simulink model "testrig_AxleTA4Watts"  (R2025b)
settings: Solver=ode23t  StartTime=0.0  StopTime=10.0  RelTol=1e-3  AbsTol=1e-3  EnableMultiTasking=on
PostLoadFcn:
  | sm_car_load_vehicle_data(bdroot,'231');
undefined symbols (not defined in the file): Vehicle, X, Y, Z
libraries: sm_lib x15, fl_lib x8, Damper_Element x2, Spring_Element x2, Susp_AxleTA4Watts x1, nesl_utility x1
Description:
  | Testrig for Solid Axle, Four Trailing Arm, Watts Link Suspension
  | 
  | Copyright 2018-2025 The MathWorks, Inc.
settings Model: VariantFading=off  Creator=smiller  LastModifiedBy=smiller
settings SolverCC: AutoScaleAbsTol=off  AlgebraicLoopSolver=TrustRegion
settings DataIOCC: LimitDataPoints=on  ReturnWorkspaceOutputs=off  SignalLoggingName=logsout_testrig_AxleTA4Watts
settings OptimizationCC: LifeSpan=inf
settings DebuggingCC: UnconnectedInputMsg=warning  UnconnectedOutputMsg=warning  UnconnectedLineMsg=warning  AllowSymbolicDim=off  SFUnexpectedBacktrackingDiag=warning  SFNoUnconditionalDefaultTransitionDiag=warning  SFExecutionAtInitializationDiag=none  ArithmeticOperatorsInVariantConditions=warning
settings ModelReferenceCC: EnableRefExpFcnMdlSchedulingChecks=on
settings SFSimCC: SimUseLocalCustomCode=off  CustomCodeUndefinedFunction=UseInterfaceOnly
settings RTWCC: RTWUseLocalCustomCode=off  GPUComputeCapability=3.5  DLArmComputeVersion=19.05
settings CodeAppCC: StateflowObjectComments=on
settings GRTTargetCC: TargetLangStandard=C89/C90 (ANSI)
settings ConfigComp: CovMetricSettings=dw  CovSaveCumulativeToWorkspaceVar=on  CovSaveSingleToWorkspaceVar=on  CovExternalEMLEnable=off  CovSFcnEnable=off
settings SimscapeCC: SimscapeNominalValues="[{\"value\":\"10\",\"unit\":\"V\"},{\"value\":\"1\",\"unit\":\"A\"},{\"value\":\"10\",\"unit\":\"N*m\"},{\"value\":\"10\",\"unit\":\"bar\"},{\"value\":\"100\",\"unit\":\"kJ/kg\"},{\"value\":\"1\",\"unit\":\"kW\"},{\"value\":\"300\",\"unit\":\"K\"},{\"value\":\"100\",\"unit\":\"cm^3/s\"},{\"value\":\"1\",\"unit\":\"kN\"},{\"value\":\"1\",\"unit\":\"g/cm^3\"},{\"value\":\"1\",\"unit\":\"l\"},{\"value\":\"1\",\"unit\":\"cm^2\"},{\"value\":\"60\",\"unit\":\"Hz\"}]"  SimscapeLogType=all  SimscapeLogName=simlog_testrig_AxleTA3  SimscapeLogLimitData=off  SimscapeLogDataHistory=10000.0
settings ConfigurationSet: Description=SimMechanics 2G
settings DiagnosticsConfigSet: SimMechanicsUnconnectedFramePorts=none  SimMechanicsConflictingReferenceFrames=none
settings ExplorerConfigSet: InternalSimMechanicsExplorerSettings="<ExplorerConfiguration><canonicalview>default</canonicalview><AnimationSetting><BasePlaybackSpeed>1.0</BasePlaybackSpeed><PlaybackSpeedFactor>1.0</PlaybackSpeedFactor></AnimationSetting><TilePanel><TileInfo><Tiles Columns=\"2\" Count=\"3\" Rows=\"2\"><Column Weight=\"0.4244\"/><Column Weight=\"0.5756\"/><Row Weight=\"0.4992\"/><Row Weight=\"0.5008\"/><Tile Height=\"2\" Width=\"1\" X=\"0\" Y=\"0\"/><Tile Height=\"1\" Width=\"1\" X=\"1\" Y=\"0\"/><Tile Height=\"1\" Width=\"1\" X=\"1\" Y=\"1\"/></Tiles></TileInfo><SceneInfo><SceneViewer><BGColor><R>1</R><G>1</G><B>1</B></BGColor><Camera><DoPerspective>off</DoPerspective><Position><X>0.552478174350915729</X><Y>-0.803945093768714147</Y><Z>1.32502797539261552</Z></Position><Center><X>0.0812867764930292336</X><Y>0.0151540971816948034</Y><Z>0.373221841276778488</Z></Center><Up><X>-0.368839640393352541</X><Y>0.60639690830076276</Y><Z>0.704443119973344745</Z></Up><ViewLimDist>1</ViewLimDist><YLim>1.05019854224089437</YLim><XLim>0.873694585561752501</XLim></Camera></SceneViewer><SceneViewer><BGColor><R>1</R><G>1</G><B>1</B></BGColor><Camera><DoPerspective>off</DoPerspective><Position><X>0.0192474230206069602</X><Y>0.00226632239327399527</Y><Z>2.4899249315669274</Z></Position><Center><X>0.0192474230206069602</X><Y>0.00226632239327399527</Y><Z>0.826695781607784674</Z></Center><Up><X>-0.999990402627246699</X><Y>-0.00438117032276797314</Y><Z>0</Z></Up><ViewLimDist>1</ViewLimDist><YLim>0.508295861926471582</YLim><XLim>1.16532602435983668</XLim></Camera></SceneViewer><SceneViewer><BGColor><R>1</R><G>1</G><B>1</B></BGColor><Camera><DoPerspective>off</DoPerspective><Position><X>0.182585918864573593</X><Y>-1.79252728458574717</Y><Z>0.406437226559380693</Z></Position><Center><X>0.182585918864573593</X><Y>0.0093803152648429533</Y><Z>0.406437226559380693</Z></Center><Up><X>0</X><Y>-0</Y><Z>1</Z></Up><ViewLimDist>1</ViewLimDist><YLim>0.57204496088982637</YLim><XLim>1.30776284260082121</XLim></Camera></SceneViewer></SceneInfo></TilePanel><MechEditorPanel><Cameras/><GfxPanelCameraMap/><VideoCreator><PlaybackSpeedRatio>1.0</PlaybackSpeedRatio><FrameRate>30</FrameRate><VideoFormat>MPEG-4</VideoFormat><FrameSize>auto</FrameSize></VideoCreator></MechEditorPanel></ExplorerConfiguration>"

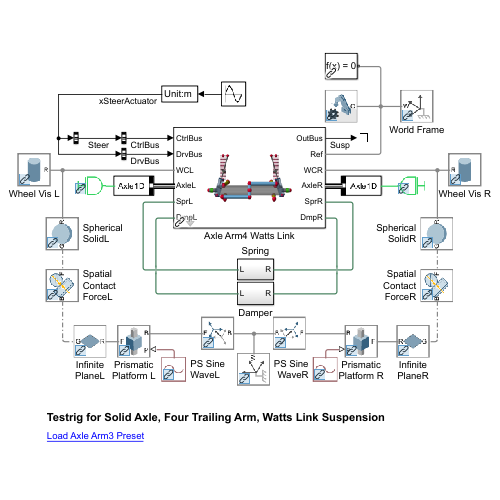
[thumbnail: Simulink's stored preview of the top-level diagram]
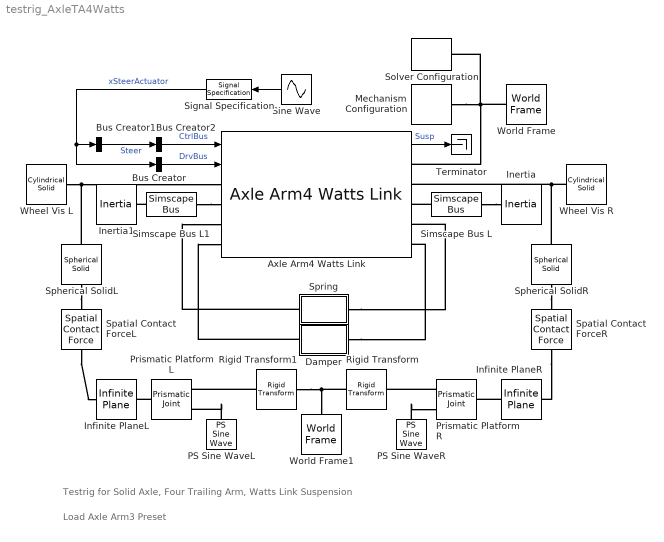
== system testrig_AxleTA4Watts ==
  note: Load Axle Arm3 Preset
  note: Testrig for Solid Axle, Four Trailing Arm, Watts Link Suspension
  Axle Arm4 Watts Link : Susp_AxleTA4Watts/Axle Arm4 Watts Link  VariantControl=LiveAxle  Init=Init.Axle2  hp_damper_top=Vehicle.Chassis.SuspA2.AxleTA4Watts.Damper.sTop.Value  hp_damper_bot=Vehicle.Chassis.SuspA2.AxleTA4Watts.Damper.sBottom.Value  hp_spring_top=Vehicle.Chassis.SuspA2.AxleTA4Watts.Spring.sTop.Value  hp_spring_bot=Vehicle.Chassis.SuspA2.AxleTA4Watts.Spring.sBottom.Value  hp_ua_body=Vehicle.Chassis.SuspA2.AxleTA4Watts.TrailingArmUpper.sBody.Value  hp_ua_axle=Vehicle.Chassis.SuspA2.AxleTA4Watts.TrailingArmUpper.sAxle.Value  hp_la_body=Vehicle.Chassis.SuspA2.AxleTA4Watts.TrailingArmLower.sBody.Value  hp_la_axle=Vehicle.Chassis.SuspA2.AxleTA4Watts.TrailingArmLower.sAxle.Value  hp_wattsu_body=Vehicle.Chassis.SuspA2.AxleTA4Watts.WattsLinkUpper.sBody.Value  hp_wattsu_pivot=Vehicle.Chassis.SuspA2.AxleTA4Watts.WattsLinkUpper.sPivot.Value  hp_wattsl_body=Vehicle.Chassis.SuspA2.AxleTA4Watts.WattsLinkLower.sBody.Value  hp_wattsl_pivot=Vehicle.Chassis.SuspA2.AxleTA4Watts.WattsLinkLower.sPivot.Value  hp_wattsp_axle=Vehicle.Chassis.SuspA2.AxleTA4Watts.WattsLinkPivot.sAxle.Value  hp_axle_cg=Vehicle.Chassis.SuspA2.AxleTA4Watts.Axle.sCG.Value  hp_whl_ctr=Vehicle.Chassis.SuspA2.AxleTA4Watts.Axle.sWheelCentre.Value  hp_chassis_bumpstop=Vehicle.Chassis.SuspA2.AxleTA4Watts.Bumpstop.sChassis.Value  hp_axle_bumpstop=Vehicle.Chassis.SuspA2.AxleTA4Watts.Bumpstop.sAxle.Value  axle_mass=Vehicle.Chassis.SuspA2.AxleTA4Watts.Axle.m.Value  stub_axle_len=Vehicle.Chassis.SuspA2.AxleTA4Watts.StubAxle.xAxle.Value  stub_axle_mass=Vehicle.Chassis.SuspA2.AxleTA4Watts.StubAxle.m.Value  axle_whlc_to_bearing=Vehicle.Chassis.SuspA2.AxleTA4Watts.Axle.xWCtoBearing.Value  ua_mass=Vehicle.Chassis.SuspA2.AxleTA4Watts.TrailingArmUpper.m.Value  la_mass=Vehicle.Chassis.SuspA2.AxleTA4Watts.TrailingArmLower.m.Value  wattsu_mass=Vehicle.Chassis.SuspA2.AxleTA4Watts.WattsLinkUpper.m.Value  wattsl_mass=Vehicle.Chassis.SuspA2.AxleTA4Watts.WattsLinkLower.m.Value  wattsp_mass=Vehicle.Chassis.SuspA2.AxleTA4Watts.WattsLinkLower.m.Value  clr_conn_rod=Visual.hp.clr  opc_conn_rod=Visual.hp.opc  size_conn_rod=Visual.hp.rad  clr_rod=Visual.UpperArm.clr  opc_rod=Visual.part.opc  radius_rod=Visual.UpperArm.rad  clr_link=Visual.Pushrod.clr  opc_link=Visual.part.opc  radius_link=Visual.Pushrod.rad  axle_clr=[0.5 0.5 0.5]  axle_opc=Visual.part.opc  clr_stub_axle=Visual.Axle.clr  opc_stub_axle=Visual.part.opc  rad_stub_axle=Visual.Axle.rad  shock_pist_mass=Vehicle.Chassis.SuspA2.AxleTA4Watts.Damper.mPiston.Value  shock_cyl_mass=Vehicle.Chassis.SuspA2.AxleTA4Watts.Damper.mCylinder.Value  shock_xmax=Vehicle.Chassis.SuspA2.AxleTA4Watts.Endstop.xMax.Value  shock_xmin=Vehicle.Chassis.SuspA2.AxleTA4Watts.Endstop.xMin.Value  spring_mass=Vehicle.Chassis.SuspA2.AxleTA4Watts.Spring.m.Value  Bumpstop_Type=Vehicle.Chassis.SuspA2.AxleTA4Watts.Bumpstop.class.Value  bumpstop_height=Vehicle.Chassis.SuspA2.AxleTA4Watts.Bumpstop.xHeight.Value  bumpstop_k=Vehicle.Chassis.SuspA2.AxleTA4Watts.Bumpstop.K.Value  bumpstop_d=Vehicle.Chassis.SuspA2.AxleTA4Watts.Bumpstop.d.Value  bumpstop_xTrans=Vehicle.Chassis.SuspA2.AxleTA4Watts.Bumpstop.xTransition.Value  bumpstop_ptcld=Vehicle.Chassis.SuspA2.AxleTA4Watts.Bumpstop.sPointCloud.Value
  Bus Creator : BusCreator  Inputs=1
  Bus Creator1 : BusCreator  Inputs=1
  Bus Creator2 : BusCreator  Inputs=1
  Damper : Subsystem
  Inertia : fl_lib/Mechanical/Rotational Elements/Inertia  inertia=1 kg*m^2  num_ports=foundation.enum.numPorts2.one  w_specify=on  w_priority=None  w=0 rad/s  w_nominal_specify=off  w_nominal_value=1  w_nominal_unit=rad/s  t_specify=off  t_priority=None  t=0 N*m  t_nominal_specify=off  t_nominal_value=1  t_nominal_unit=N*m
  Inertia1 : fl_lib/Mechanical/Rotational Elements/Inertia  inertia=1 kg*m^2  num_ports=foundation.enum.numPorts2.one  w_specify=on  w_priority=None  w=0 rad/s  w_nominal_specify=off  w_nominal_value=1  w_nominal_unit=rad/s  t_specify=off  t_priority=None  t=0 N*m  t_nominal_specify=off  t_nominal_value=1  t_nominal_unit=N*m
  Infinite PlaneL : sm_lib/Curves and Surfaces/Infinite Plane  GraphicType=Rectangle  GraphicPlaneWidth=0.3  GraphicPlaneWidthUnits=m  GraphicPlaneHeight=0.3  GraphicPlaneHeightUnits=m  GraphicVisPropType=SimpleVisualProperties  GraphicDiffuseColor=[0.5 0.5 0.5]  GraphicOpacity=0.5  GraphicSpecularColor=[0.5 0.5 0.5 1.0]  GraphicAmbientColor=[0.15 0.15 0.15 1.0]  GraphicEmissiveColor=[0.0 0.0 0.0 1.0]  GraphicShininess=75
  Infinite PlaneR : sm_lib/Curves and Surfaces/Infinite Plane  GraphicType=Rectangle  GraphicPlaneWidth=0.3  GraphicPlaneWidthUnits=m  GraphicPlaneHeight=0.3  GraphicPlaneHeightUnits=m  GraphicVisPropType=SimpleVisualProperties  GraphicDiffuseColor=[0.5 0.5 0.5]  GraphicOpacity=0.5  GraphicSpecularColor=[0.5 0.5 0.5 1.0]  GraphicAmbientColor=[0.15 0.15 0.15 1.0]  GraphicEmissiveColor=[0.0 0.0 0.0 1.0]  GraphicShininess=75
  Mechanism Configuration : sm_lib/Utilities/Mechanism Configuration  UniformGravity=Constant  GravityVector=[0 0 -9.80665]  GravityVectorUnits=m/s^2  LinearizationDelta=0.001  JointModeTransitionNonlinearIterations=2
  PS Sine WaveL : fl_lib/Physical Signals/Sources/PS Sine Wave  amplitude=0.05 m  bias=0 m  frequency_spec=foundation.enum.frequencySpec.frequencySI  frequency_SI=4/3 Hz  frequency_angular=1 rad/s  phase=pi rad
      settings: InternalSimscapePortConfiguration="{\"Bottom\":[],\"Left\":[],\"Right\":[{\"id\":\"O\",\"label\":\"\",\"type\":\"output\"}],\"Top\":[]}"
  PS Sine WaveR : fl_lib/Physical Signals/Sources/PS Sine Wave  amplitude=0.1 m  bias=0 m  frequency_spec=foundation.enum.frequencySpec.frequencySI  frequency_SI=1 Hz  frequency_angular=1 rad/s  phase=0 rad
      settings: InternalSimscapePortConfiguration="{\"Bottom\":[],\"Left\":[],\"Right\":[{\"id\":\"O\",\"label\":\"\",\"type\":\"output\"}],\"Top\":[]}"
  Prismatic Platform L : sm_lib/Joints/Prismatic Joint  JointMode=Normal  CompositeWrenchDir=FollowerOnBase  CompositeWrenchFrame=BaseFrame  SenseConstraintForce=off  SenseConstraintTorque=off  SenseTotalForce=off  SenseTotalTorque=off  PositionTargetSpecify=off  PositionTargetPriority=High  PositionTargetValue=0  PositionTargetValueUnits=m  VelocityTargetSpecify=off  VelocityTargetPriority=High  VelocityTargetValue=0  VelocityTargetValueUnits=m/s  EquilibriumPosition=0  EquilibriumPositionUnits=m  SpringStiffness=0  SpringStiffnessUnits=N/m  DampingCoefficient=0  DampingCoefficientUnits=N/(m/s)  LowerLimitSpecify=off  LowerLimitBound=-1  LowerLimitBoundUnits=m  LowerLimitStiffness=1e6  LowerLimitStiffnessUnits=N/m  LowerLimitDamping=1e3  LowerLimitDampingUnits=N/(m/s)  LowerLimitTransitionRegionWidth=1e-4  LowerLimitTransitionRegionWidthUnits=m  UpperLimitSpecify=off  UpperLimitBound=1  UpperLimitBoundUnits=m  UpperLimitStiffness=1e6  UpperLimitStiffnessUnits=N/m  UpperLimitDamping=1e3  UpperLimitDampingUnits=N/(m/s)  UpperLimitTransitionRegionWidth=1e-4  UpperLimitTransitionRegionWidthUnits=m  TorqueActuationMode=ComputedTorque  MotionActuationMode=InputMotion  SensePosition=off  SenseVelocity=off  SenseAcceleration=off  SenseTorqueForce=off  SenseLowerLimitTorqueForce=off  SenseUpperLimitTorqueForce=off
  Prismatic Platform R : sm_lib/Joints/Prismatic Joint  JointMode=Normal  CompositeWrenchDir=FollowerOnBase  CompositeWrenchFrame=BaseFrame  SenseConstraintForce=off  SenseConstraintTorque=off  SenseTotalForce=off  SenseTotalTorque=off  PositionTargetSpecify=off  PositionTargetPriority=High  PositionTargetValue=0  PositionTargetValueUnits=m  VelocityTargetSpecify=off  VelocityTargetPriority=High  VelocityTargetValue=0  VelocityTargetValueUnits=m/s  EquilibriumPosition=0  EquilibriumPositionUnits=m  SpringStiffness=0  SpringStiffnessUnits=N/m  DampingCoefficient=0  DampingCoefficientUnits=N/(m/s)  LowerLimitSpecify=off  LowerLimitBound=-1  LowerLimitBoundUnits=m  LowerLimitStiffness=1e6  LowerLimitStiffnessUnits=N/m  LowerLimitDamping=1e3  LowerLimitDampingUnits=N/(m/s)  LowerLimitTransitionRegionWidth=1e-4  LowerLimitTransitionRegionWidthUnits=m  UpperLimitSpecify=off  UpperLimitBound=1  UpperLimitBoundUnits=m  UpperLimitStiffness=1e6  UpperLimitStiffnessUnits=N/m  UpperLimitDamping=1e3  UpperLimitDampingUnits=N/(m/s)  UpperLimitTransitionRegionWidth=1e-4  UpperLimitTransitionRegionWidthUnits=m  TorqueActuationMode=ComputedTorque  MotionActuationMode=InputMotion  SensePosition=off  SenseVelocity=off  SenseAcceleration=off  SenseTorqueForce=off  SenseLowerLimitTorqueForce=off  SenseUpperLimitTorqueForce=off
  Rigid Transform : sm_lib/Frames and Transforms/Rigid Transform  RotationMethod=None  FollAlignAxisA=+X  BaseAlignAxisA=+Y  FollAlignAxisB=+Y  BaseAlignAxisB=+Z  RotationStandardAxis=+Z  RotationAngle=0  RotationAngleUnits=deg  RotationArbitraryAxis=[0 0 1]  RotationSequenceAxes=FollowerAxes  RotationSequence=XYX  RotationSequenceAngles=[0 0 0]  RotationSequenceAnglesUnits=deg  RotationMatrix=[1 0 0;0 1 0;0 0 1]  Quaternion=[1 0 0 0]  TranslationMethod=Cartesian  TranslationCartesianOffset=Vehicle.Chassis.SuspA2.AxleTA4Watts.Axle.sWheelCentre.Value.*[1 -1 0]  TranslationCartesianOffsetUnits=m  TranslationStandardAxis=+Z  TranslationStandardOffset=0  TranslationStandardOffsetUnits=m  TranslationROffset=0  TranslationROffsetUnits=m  TranslationThetaOffset=0  TranslationThetaOffsetUnits=deg  TranslationZOffset=0  TranslationZOffsetUnits=m
  Rigid Transform1 : sm_lib/Frames and Transforms/Rigid Transform  RotationMethod=None  FollAlignAxisA=+X  BaseAlignAxisA=+Y  FollAlignAxisB=+Y  BaseAlignAxisB=+Z  RotationStandardAxis=+Z  RotationAngle=0  RotationAngleUnits=deg  RotationArbitraryAxis=[0 0 1]  RotationSequenceAxes=FollowerAxes  RotationSequence=XYX  RotationSequenceAngles=[0 0 0]  RotationSequenceAnglesUnits=deg  RotationMatrix=[1 0 0;0 1 0;0 0 1]  Quaternion=[1 0 0 0]  TranslationMethod=Cartesian  TranslationCartesianOffset=Vehicle.Chassis.SuspA2.AxleTA4Watts.Axle.sWheelCentre.Value.*[1 1 0]  TranslationCartesianOffsetUnits=m  TranslationStandardAxis=+Z  TranslationStandardOffset=0  TranslationStandardOffsetUnits=m  TranslationROffset=0  TranslationROffsetUnits=m  TranslationThetaOffset=0  TranslationThetaOffsetUnits=deg  TranslationZOffset=0  TranslationZOffsetUnits=m
  Signal Specification : SignalSpecification  Unit=m
  Simscape Bus L : SimscapeBus  HierarchyStrings=Axle1D
  Simscape Bus L1 : SimscapeBus  HierarchyStrings=Axle1D
  Sine Wave : Sin  Amplitude=0.1  Frequency=pi/4  SampleTime=0
  Solver Configuration : nesl_utility/Solver Configuration  PhysicalDomain=network_engine_domain  SubClassName=solver  LeftPortType=input  RightPortType=generic  Tones=[]  Harmonics=[]  SimulateNoise=off  Profile=off  UseLocalSampling=off  EnableSwitchedLinearOptims=on  FrequencyDomain=off  UseCCode=off  RelTol=0.001  AbsTol=1e-06  MinStep=1e-09  ToWorkspace=off  RevertToSquareIcSolve=off  NumHomotopyIterations=100  PhasorMode=off  PhasorModeNumHarmonics=1  ConsistencySolver=NEWTON_FTOL  IndexReductionMethod=DerivativeReplacement  DoDC=off  ResidualTolerance=1e-09  ConsistencyTolSource=GLOBAL  ConsistencyAbsTol=0.001  ConsistencyRelTol=0.001  ConsistencyTolFactor=0.001  UseLocalSolver=off  LocalSolverChoice=NE_BACKWARD_EULER_ADVANCER  ResolveIndetEquations=on  FunctionEvalNumThread=1  LocalSolverSampleTime=0.001  DoFixedCost=off  MaxNonlinIter=3  MaxModeIter=2  ComputeImpulses=off  ImpulseIterations=2  LinearAlgebra=Sparse  LinearAlgebraNumThread=0  EquationFormulation=NE_TIME_EF  DelaysMemoryBudget=1024  AutomaticFiltering=on  FilteringTimeConstant=0.001  PartitionStorageMethod=AS_NEEDED  PartitionMemoryBudget=1024  PartitionMethod=FAST  MultibodyUseLocalSolver=off  MultibodyLocalSolverChoice=ODE1  MultibodyLocalSolverSampleTime=0.001
  Spatial Contact ForceL : sm_lib/Forces and Torques/Spatial Contact Force  SenseSeparationDistance=off  NormalForceType=SmoothSpringDamper  NormalStiffness=1e6  NormalStiffnessUnits=N/m  NormalDamping=1e3  NormalDampingUnits=N/(m/s)  NormalTransitionRegionWidth=1e-4  NormalTransitionRegionWidthUnits=m  FrictionType=None  CoefficientOfStaticFriction=0.5  CoefficientOfDynamicFriction=0.3  FrictionalCriticalVelocity=1e-3  FrictionalCriticalVelocityUnits=m/s  SenseContactSignal=off  SensePenetrationDepth=off  SenseNormalVelocity=off  SenseTangentialVelocity=off  SensingForceTorqueDirection=BaseOnFollower  SensingForceTorqueResolutionFrame=ContactFrame  SenseNormalForce=off  SenseNormalForceMagnitude=off  SenseNormalTorque=off  SenseFrictionalForce=off  SenseFrictionalForceMagnitude=off  SenseFrictionalTorque=off  SenseTotalForce=off  SenseTotalTorque=off  SenseContactBaseRotation=off  SenseContactBaseTranslation=off  SenseContactFollowerRotation=off  SenseContactFollowerTranslation=off  ZeroCrossDetectContactStartAndEnd=off
  Spatial Contact ForceR : sm_lib/Forces and Torques/Spatial Contact Force  SenseSeparationDistance=off  NormalForceType=SmoothSpringDamper  NormalStiffness=1e6  NormalStiffnessUnits=N/m  NormalDamping=1e3  NormalDampingUnits=N/(m/s)  NormalTransitionRegionWidth=1e-4  NormalTransitionRegionWidthUnits=m  FrictionType=None  CoefficientOfStaticFriction=0.5  CoefficientOfDynamicFriction=0.3  FrictionalCriticalVelocity=1e-3  FrictionalCriticalVelocityUnits=m/s  SenseContactSignal=off  SensePenetrationDepth=off  SenseNormalVelocity=off  SenseTangentialVelocity=off  SensingForceTorqueDirection=BaseOnFollower  SensingForceTorqueResolutionFrame=ContactFrame  SenseNormalForce=off  SenseNormalForceMagnitude=off  SenseNormalTorque=off  SenseFrictionalForce=off  SenseFrictionalForceMagnitude=off  SenseFrictionalTorque=off  SenseTotalForce=off  SenseTotalTorque=off  SenseContactBaseRotation=off  SenseContactBaseTranslation=off  SenseContactFollowerRotation=off  SenseContactFollowerTranslation=off  ZeroCrossDetectContactStartAndEnd=off
  Spherical SolidL : sm_lib/Body Elements/Spherical Solid  SphereRadius=Vehicle.Chassis.SuspA2.AxleTA4Watts.Axle.sWheelCentre.Value(3)  SphereRadiusUnits=m  ExportEntireGeometry=on  InertiaType=CalculateFromGeometry  BasedOnType=Density  Density=0  DensityUnits=kg/m^3  Mass=1  MassUnits=kg  CenterOfMass=[0 0 0]  CenterOfMassUnits=m  MomentsOfInertia=[1 1 1]  MomentsOfInertiaUnits=kg*m^2  ProductsOfInertia=[0 0 0]  ProductsOfInertiaUnits=kg*m^2  GraphicType=None  MarkerShape=Sphere  MarkerSize=10  GraphicVisPropType=SimpleVisualProperties  GraphicDiffuseColor=[1.0 0.0 0.2]  GraphicOpacity=0.5  GraphicSpecularColor=[0.5 0.5 0.5 1.0]  GraphicAmbientColor=[0.15 0.15 0.15 1.0]  GraphicEmissiveColor=[0.0 0.0 0.0 1.0]  GraphicShininess=75  DoExposeReferenceFrame=on  SerializedFrames=<Frames/>
  Spherical SolidR : sm_lib/Body Elements/Spherical Solid  SphereRadius=Vehicle.Chassis.SuspA2.AxleTA4Watts.Axle.sWheelCentre.Value(3)  SphereRadiusUnits=m  ExportEntireGeometry=on  InertiaType=CalculateFromGeometry  BasedOnType=Density  Density=0  DensityUnits=kg/m^3  Mass=1  MassUnits=kg  CenterOfMass=[0 0 0]  CenterOfMassUnits=m  MomentsOfInertia=[1 1 1]  MomentsOfInertiaUnits=kg*m^2  ProductsOfInertia=[0 0 0]  ProductsOfInertiaUnits=kg*m^2  GraphicType=None  MarkerShape=Sphere  MarkerSize=10  GraphicVisPropType=SimpleVisualProperties  GraphicDiffuseColor=[1.0 0.0 0.2]  GraphicOpacity=0.5  GraphicSpecularColor=[0.5 0.5 0.5 1.0]  GraphicAmbientColor=[0.15 0.15 0.15 1.0]  GraphicEmissiveColor=[0.0 0.0 0.0 1.0]  GraphicShininess=75  DoExposeReferenceFrame=on  SerializedFrames=<Frames/>
  Spring : Subsystem
  Terminator : Terminator
  Wheel Vis L : sm_lib/Body Elements/Cylindrical Solid  CylinderRadius=Vehicle.Chassis.SuspA2.AxleTA4Watts.Axle.sWheelCentre.Value(3)  CylinderRadiusUnits=m  CylinderLength=0.235  CylinderLengthUnits=m  ExportEntireGeometry=off  InertiaType=CalculateFromGeometry  BasedOnType=Density  Density=1000  DensityUnits=kg/m^3  Mass=1  MassUnits=kg  CenterOfMass=[0 0 0]  CenterOfMassUnits=m  MomentsOfInertia=[1 1 1]  MomentsOfInertiaUnits=kg*m^2  ProductsOfInertia=[0 0 0]  ProductsOfInertiaUnits=kg*m^2  GraphicType=FromGeometry  MarkerShape=Sphere  MarkerSize=10  GraphicVisPropType=SimpleVisualProperties  GraphicDiffuseColor=[0.5 0.5 0.5]  GraphicOpacity=0.3  GraphicSpecularColor=[0.5 0.5 0.5 1.0]  GraphicAmbientColor=[0.15 0.15 0.15 1.0]  GraphicEmissiveColor=[0.0 0.0 0.0 1.0]  GraphicShininess=75  DoExposeReferenceFrame=on  SerializedFrames=<Frames/>
  Wheel Vis R : sm_lib/Body Elements/Cylindrical Solid  CylinderRadius=Vehicle.Chassis.SuspA2.AxleTA4Watts.Axle.sWheelCentre.Value(3)  CylinderRadiusUnits=m  CylinderLength=0.235  CylinderLengthUnits=m  ExportEntireGeometry=off  InertiaType=CalculateFromGeometry  BasedOnType=Density  Density=1000  DensityUnits=kg/m^3  Mass=1  MassUnits=kg  CenterOfMass=[0 0 0]  CenterOfMassUnits=m  MomentsOfInertia=[1 1 1]  MomentsOfInertiaUnits=kg*m^2  ProductsOfInertia=[0 0 0]  ProductsOfInertiaUnits=kg*m^2  GraphicType=FromGeometry  MarkerShape=Sphere  MarkerSize=10  GraphicVisPropType=SimpleVisualProperties  GraphicDiffuseColor=[0.5 0.5 0.5]  GraphicOpacity=0.3  GraphicSpecularColor=[0.5 0.5 0.5 1.0]  GraphicAmbientColor=[0.15 0.15 0.15 1.0]  GraphicEmissiveColor=[0.0 0.0 0.0 1.0]  GraphicShininess=75  DoExposeReferenceFrame=on  SerializedFrames=<Frames/>
  World Frame : sm_lib/Frames and Transforms/World Frame
  World Frame1 : sm_lib/Frames and Transforms/World Frame
  wires:
  Sine Wave/1 -> Signal Specification/1
  Signal Specification/1 -> Bus Creator/1, Bus Creator1/1  "xSteerActuator"
  Bus Creator/1 -> Axle Arm4 Watts Link/2  "DrvBus"
  Bus Creator1/1 -> Bus Creator2/1  "Steer"
  Axle Arm4 Watts Link/1 -> Terminator/1  "Susp"
  Bus Creator2/1 -> Axle Arm4 Watts Link/1  "CtrlBus"
  connections:
  Wheel Vis L/RConn1 -- Spherical SolidL/RConn1 -- Axle Arm4 Watts Link/LConn1
  Simscape Bus L/LConn1 -- Inertia/LConn1
  Simscape Bus L1/LConn1 -- Inertia1/LConn1
  Wheel Vis R/RConn1 -- Spherical SolidR/RConn1 -- Axle Arm4 Watts Link/RConn2
  Spherical SolidR/LConn1 -- Spatial Contact ForceR/RConn1
  Rigid Transform/LConn1 -- Rigid Transform1/LConn1 -- World Frame1/RConn1
  Spherical SolidL/LConn1 -- Spatial Contact ForceL/RConn1
  Spatial Contact ForceR/LConn1 -- Infinite PlaneR/RConn1
  Spatial Contact ForceL/LConn1 -- Infinite PlaneL/RConn1
  Infinite PlaneR/LConn1 -- Prismatic Platform R/RConn1
  Prismatic Platform L/RConn1 -- Infinite PlaneL/LConn1
  PS Sine WaveR/RConn1 -- Prismatic Platform R/LConn2
  PS Sine WaveL/RConn1 -- Prismatic Platform L/LConn2
  Prismatic Platform R/LConn1 -- Rigid Transform/RConn1
  Rigid Transform1/RConn1 -- Prismatic Platform L/LConn1
  Mechanism Configuration/RConn1 -- Axle Arm4 Watts Link/RConn1 -- Solver Configuration/RConn1 -- World Frame/RConn1
  Simscape Bus L1/RConn1 -- Axle Arm4 Watts Link/LConn2
  Simscape Bus L/RConn1 -- Axle Arm4 Watts Link/RConn3
  Spring/LConn1 -- Axle Arm4 Watts Link/LConn3
  Spring/RConn1 -- Axle Arm4 Watts Link/RConn4
  Damper/LConn1 -- Axle Arm4 Watts Link/LConn4
  Damper/RConn1 -- Axle Arm4 Watts Link/RConn5

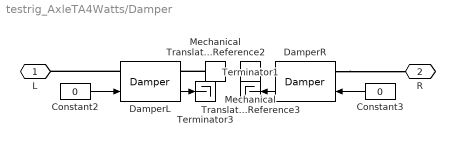
== system testrig_AxleTA4Watts/Damper ==
  Constant2 : Constant  Value=0
  Constant3 : Constant  Value=0
  DamperL : Damper_Element/Damper  VariantControl=Variant1  LabelModeActiveChoice=Linear  Damper=Vehicle.Chassis.Damper.Axle1  VariantLabel=Vehicle.Chassis.Damper.Axle1.class.Value
      settings: AttributesFormatString=%<ActiveVariant>
  DamperR : Damper_Element/Damper  VariantControl=Variant1  LabelModeActiveChoice=Linear  Damper=Vehicle.Chassis.Damper.Axle1  VariantLabel=Vehicle.Chassis.Damper.Axle1.class.Value
      settings: AttributesFormatString=%<ActiveVariant>
  Mechanical Translational Reference2 : fl_lib/Mechanical/Translational Elements/Mechanical Translational Reference
  Mechanical Translational Reference3 : fl_lib/Mechanical/Translational Elements/Mechanical Translational Reference
  Terminator1 : Terminator
  Terminator3 : Terminator
  L : PMIOPort  Side=Left
  R : PMIOPort  Port=2  Side=Right
  wires:
  DamperR/1 -> Terminator1/1
  Constant3/1 -> DamperR/1
  Constant2/1 -> DamperL/1
  DamperL/1 -> Terminator3/1
  connections:
  DamperL/LConn1 -- L/RConn1
  Mechanical Translational Reference2/LConn1 -- DamperL/RConn1
  Mechanical Translational Reference3/LConn1 -- DamperR/RConn1
  DamperR/LConn1 -- R/RConn1

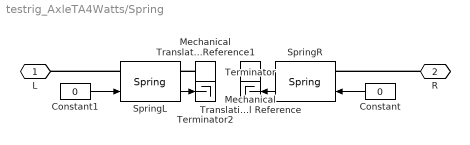
== system testrig_AxleTA4Watts/Spring ==
  Constant : Constant  Value=0
  Constant1 : Constant  Value=0
  Mechanical Translational Reference : fl_lib/Mechanical/Translational Elements/Mechanical Translational Reference
  Mechanical Translational Reference1 : fl_lib/Mechanical/Translational Elements/Mechanical Translational Reference
  SpringL : Spring_Element/Spring  VariantControl=Variant1  LabelModeActiveChoice=Linear  Spring=Vehicle.Chassis.Spring.Axle1  VariantLabel=Vehicle.Chassis.Spring.Axle1.class.Value
      settings: AttributesFormatString=%<ActiveVariant>
  SpringR : Spring_Element/Spring  VariantControl=Variant1  LabelModeActiveChoice=Linear  Spring=Vehicle.Chassis.Spring.Axle1  VariantLabel=Vehicle.Chassis.Spring.Axle1.class.Value
      settings: AttributesFormatString=%<ActiveVariant>
  Terminator : Terminator
  Terminator2 : Terminator
  L : PMIOPort  Side=Left
  R : PMIOPort  Port=2  Side=Right
  wires:
  SpringL/1 -> Terminator2/1
  Constant1/1 -> SpringL/1
  SpringR/1 -> Terminator/1
  Constant/1 -> SpringR/1
  connections:
  Mechanical Translational Reference1/LConn1 -- SpringL/RConn1
  Mechanical Translational Reference/LConn1 -- SpringR/RConn1
  R/RConn1 -- SpringR/LConn1
  SpringL/LConn1 -- L/RConn1
